simulink model "test_function"  (R2025a)
settings: Solver=ode4  StartTime=0.0  StopTime=100  FixedStep=0.01  RelTol=1e-3
libraries: slpidlib x1
settings Model: Creator=hannasennero  LastModifiedBy=hannasennero

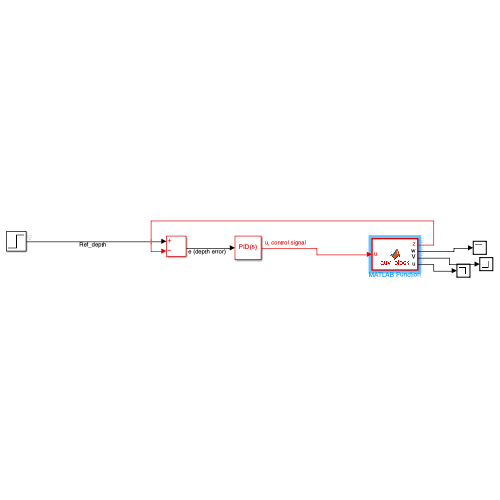
[thumbnail: Simulink's stored preview of the top-level diagram]
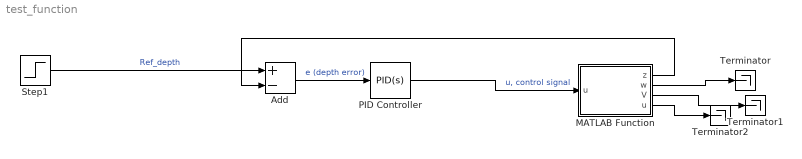
== system test_function ==
  Add : Sum  Inputs=+-
  MATLAB Function : MATLAB Function  TreatAsAtomicUnit=on
  PID Controller : slpidlib/PID Controller  Controller=PID  Form=Parallel  TimeDomain=Continuous-time  UseExternalTs=off  SampleTime=-1  IntegratorMethod=Forward Euler  FilterMethod=Forward Euler  ControllerParametersSource=internal  P=10  I=0.1  UseKiTs=off  D=5  UseExternalDerivativeSource=off  N=100  UseFilter=on  TunerSelectOption=Transfer Function Based (PID Tuner App)  InitialConditionSource=internal  InitialConditionForIntegrator=0  InitialConditionForFilter=0  DifferentiatorICPrevScaledInput=0  ExternalReset=none  TrackingMode=off  Kt=1  LimitOutput=off  SatLimitsSource=internal  UpperSaturationLimit=inf  LowerSaturationLimit=-inf  LinearizeAsGain=on  AntiWindupMode=none  Kb=1  LimitIntegrator=off  UpperIntegratorSaturationLimit=inf  LowerIntegratorSaturationLimit=-inf  POutMin=[]  POutMax=[]  IOutMin=[]  IOutMax=[]  DOutMin=[]  DOutMax=[]  NOutMin=[]  NOutMax=[]  SumOutMin=[]  SumOutMax=[]  SaturationOutMin=[]  SaturationOutMax=[]  PParamMin=[]  PParamMax=[]  IParamMin=[]  IParamMax=[]  DParamMin=[]  DParamMax=[]  NParamMin=[]  NParamMax=[]  KbParamMin=[]  KbParamMax=[]  KtParamMin=[]  KtParamMax=[]  KbOutMin=[]  KbOutMax=[]  KtOutMin=[]  KtOutMax=[]  IntegratorOutMin=[]  IntegratorOutMax=[]  FilterOutMin=[]  FilterOutMax=[]  SumI1OutMin=[]  SumI1OutMax=[]  SumI2OutMin=[]  SumI2OutMax=[]  SumI3OutMin=[]  SumI3OutMax=[]  SumI4OutMin=[]  SumI4OutMax=[]  SumDOutMin=[]  SumDOutMax=[]  DifferentiatorOutMin=[]  DifferentiatorOutMax=[]  FilterDiffOutCoefMin=[]  FilterDiffOutCoefMax=[]  ReciprocalOutMin=[]  ReciprocalOutMax=[]  SumDenOutMin=[]  SumDenOutMax=[]  SumNumOutMin=[]  SumNumOutMax=[]  DivideOutMin=[]  DivideOutMax=[]  UdiffTsProdOutMin=[]  UdiffTsProdOutMax=[]  NTsProdOutMin=[]  NTsProdOutMax=[]  UintegralTsProdOutMin=[]  UintegralTsProdOutMax=[]  UngainTsProdOutMin=[]  UngainTsProdOutMax=[]  ClampingZeroOutDataTypeStr=Inherit: Inherit via back propagation  ClampingZeroOutMin=[]  ClampingZeroOutMax=[]  FilterDenConstantOutDataTypeStr=Inherit: Inherit via back propagation  FilterDenConstantOutMin=[]  FilterDenConstantOutMax=[]  PCopyOutDataTypeStr=Inherit: Inherit via back propagation  PCopyOutMin=[]  PCopyOutMax=[]  NCopyOutDataTypeStr=Inherit: Inherit via back propagation  NCopyOutMin=[]  NCopyOutMax=[]  IntegratorContinuousStateAttributes=''  IntegratorStateMustResolveToSignalObject=off  IntegratorRTWStateStorageClass=Auto  FilterContinuousStateAttributes=''  FilterStateMustResolveToSignalObject=off  FilterRTWStateStorageClass=Auto  ParallelPVariant=InternalParameters  IdealPVariant=Disabled  IVariant=InternalParameters  DVariant=InternalParameters  IntegratorVariant=Continuous  SatVariant=Disabled  AWVariant=Passthrough  PCopyVariant=Disabled  TRVariant=Disabled  FdbkBlocksVariant=Forward  IdealPFdbkVariant=Disabled  SatFdbkVariant=Disabled  DerivativeFilterVariant=ContFilter  NVariant=InternalParameters  NCopyVariant=Disabled  FilterICVariant=InternalICsFilter  IntegratorICVariant=InternalICs  ExternalResetVariant=Disabled  TRSumVariant=Passthrough  SumFdbkVariant=Disabled  SumVariant=Sum_PID  TsampFilterVariant=InternalTs  TsampNgainVariant=Passthrough  TsampIntegralVariant=Disabled_SignalSpec  ExternalSaturationOutDataTypeStr=Inherit: Same as second input  DerivativeSourceVariant=ErrorSignal  PreIntVariant=InternalPreInt
  Step1 : Step  After=5  SampleTime=0
  Terminator : Terminator
  Terminator1 : Terminator
  Terminator2 : Terminator
  wires:
  Step1/1 -> Add/1  "Ref_depth"
  PID Controller/1 -> MATLAB Function/1("u ")  "u, control signal"
  Add/1 -> PID Controller/1  "e (depth error)"
  MATLAB Function/1(z) -> Add/2
  MATLAB Function/2(w) -> Terminator/1
  MATLAB Function/3(V) -> Terminator1/1
  MATLAB Function/4(u) -> Terminator2/1

== matlab function test_function/MATLAB Function ==
  data: u input; z output; w output; V output; u output
function [z, w, V, u] = auv_block(u)
% AUV Depth Control Model for Simulink MATLAB Function Block
% INPUTS:
%   z_ref : referensdjup (m)
%   dt    : tidssteg (s)
% OUTPUTS:
%   z     : aktuellt djup (m)
%   w     : hastighet (m/s)
%   V     : ballastvolym (m^3)
%   u     : PID-styrsignal

%% --- Parametrar (persistent så de initieras en gång) ---
persistent m g rho F_pos V_max k_m p A A_utlopp m_a C_d A_cross ...
           motor_torque F_motor_max R_flow dt P_atm
persistent z_prev w_prev V_prev t_prev

if isempty(m)
    % Farkost
    m = 3; g = 9.81; rho = 1000;
    % Buoyancy
    F_pos = 2.94 + m*g;
    V_max = 0.0005;            % 500 ml
    % Aktuator
    k_m = 5; p = 0.002; d = 0.1; A = pi*(d/2)^2; A_utlopp = pi*(0.01/2)^2;
    motor_torque = 0.65; 
    F_motor_max = 2*pi*motor_torque/p;
    % Dynamik
    m_a = 2.5; C_d = 1.0; A_cross = 0.07;
    R_flow = 1e5; P_atm = 101325;
    % Initialtillstånd
    z_prev = 0; w_prev = 0; V_prev = 0;
    dt = 0.01;
end

%% --- PID-regulator ---
max_u = 1e-4/k_m/p/A;
u = max(min(u, max_u), -max_u);

% --- Aktuator (enkel modell) ---
    V_dot = k_m * u * p * A;        % Flöde in/ur syringe

    % % % Hydrostatiskt tryck på djup z
    P_hydro = rho * g * z_prev + P_atm
    
    % % Tryck som motorn kan generera
    F_motor = F_motor_max * u;  % 0.6 = verkningsgrad
    P_motor = F_motor / A
    % 
    % Begränsa flöde baserat på tryckskillnad
    if P_motor > P_hydro && u > 0  % Pumpa in vatten
        %V_dot = V_dot * (1 - min(1, (P_hydro - P_atm) / (P_motor - P_atm)));
    elseif u <= 0  % Pumpa ut vatten (lättare på djup)
        V_dot = V_dot;
    else
        V_dot = 0;
    end

    %Strömningsmotstånd i slangar och ventiler
    delta_P_required = R_flow * abs(V_dot);
    if abs(P_motor - P_hydro) < delta_P_required
        V_dot = 0;  % Inte tillräckligt med tryck för att övervinna motståndet
    end
    V = V_prev + V_dot * dt;
    V = max(min(V, V_max), 0);      % Begränsa volym; 
    
    % --- Buoyancy ---
    F_b = rho*g*V + m*g - F_pos;    % Netto flytkraft (positiv = uppåt)
    
    % --- Hydrodynamik ---
    D = 0.5 * rho * C_d * A_cross * abs(w_prev) * w_prev;
    
    % --- Rörelseekvation ---
    F_net = F_b - D;
    m_eff = m + m_a;
    w_dot = F_net / m_eff;              % acceleration
    w = w_prev + w_dot * dt;
    
    % --- Ythantering ---
    if z_prev <= 0 && w < 0
        w = 0;
        z_prev = 0;
        %V = V_innan;
    end
    
    % --- Uppdatera position ---
    z = z_prev + w * dt;
    z = max(z, 0);

%% --- Uppdatera persistent tillstånd ---
z_prev = z; w_prev = w; V_prev = V;

end
